simulink model "COHERENT_DEMODULATOR"  (R2021b)
settings: Solver=VariableStepAuto  StartTime=0.0  StopTime=0.002  RelTol=1e-3
libraries: simulink x3, commfilt2 x2, dspsigops x2, dspsrcs4 x2
settings Model: Creator=caccolillo  LastModifiedBy=caccolillo

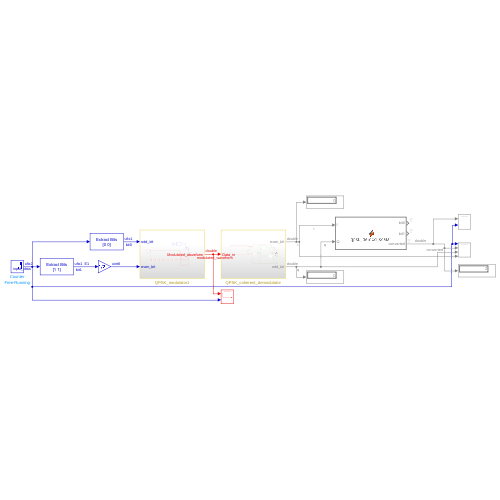
[thumbnail: Simulink's stored preview of the top-level diagram]
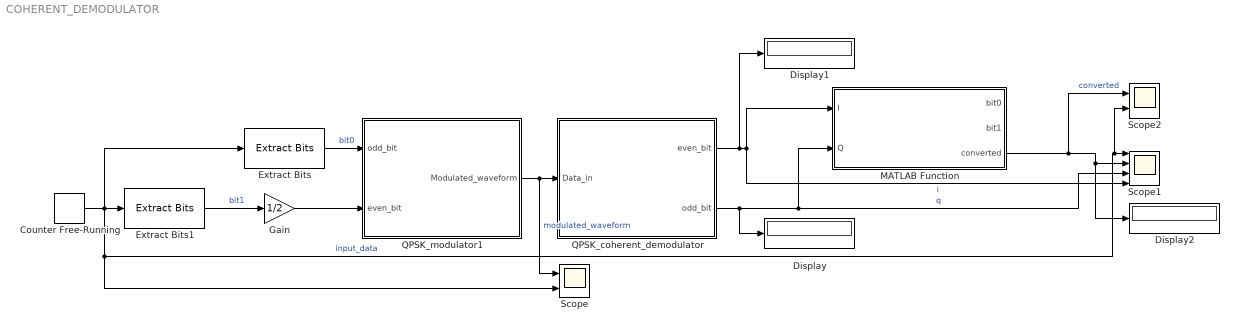
== system COHERENT_DEMODULATOR ==
  Counter Free-Running : simulink/Sources/Counter Free-Running  NumBits=2  tsamp=1/20000
  Display : Display
  Display1 : Display
  Display2 : Display
  Extract Bits : simulink/Logic and Bit Operations/Extract Bits  bitsToExtract=Range of bits  numBits=8  bitIdxRange=[0 0]  outScalingMode=Preserve fixed-point scaling
  Extract Bits1 : simulink/Logic and Bit Operations/Extract Bits  bitsToExtract=Range of bits  numBits=8  bitIdxRange=[1 1]  outScalingMode=Preserve fixed-point scaling
  Gain : Gain  Gain=1/2
  MATLAB Function : MATLAB Function  TreatAsAtomicUnit=on
  QPSK_coherent_demodulator : Subsystem
  QPSK_modulator1 : Subsystem
  Scope : Scope  NumInputPorts=2
  Scope1 : Scope  NumInputPorts=4
  Scope2 : Scope  NumInputPorts=2
  wires:
  QPSK_modulator1/1(Modulated_waveform) -> QPSK_coherent_demodulator/1(Data_in), Scope/1  "modulated_waveform"
  Counter Free-Running/1 -> Scope2/2, Scope1/1, Scope/2, Extract Bits/1, Extract Bits1/1  "input_data"
  QPSK_coherent_demodulator/2(odd_bit) -> MATLAB Function/2(Q), Scope1/3, Display/1  "q"
  QPSK_coherent_demodulator/1(even_bit) -> MATLAB Function/1(I), Scope1/4, Display1/1  "i"
  Gain/1 -> QPSK_modulator1/2(even_bit)
  MATLAB Function/3(converted) -> Scope2/1, Display2/1, Scope1/2  "converted"
  Extract Bits/1 -> QPSK_modulator1/1(odd_bit)  "bit0"
  Extract Bits1/1 -> Gain/1  "bit1"

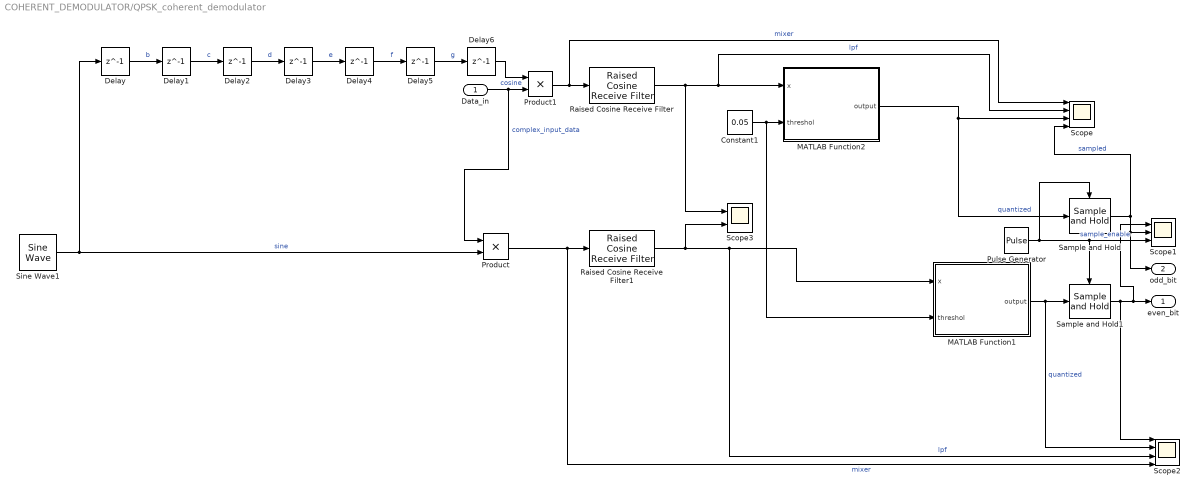
== system COHERENT_DEMODULATOR/QPSK_coherent_demodulator ==
  Data_in : Inport
  Constant1 : Constant  Value=0.05
  Delay{,1..6} (7 alike) : Delay  DelayLength=1  InitialCondition=0
  MATLAB Function1 : MATLAB Function  TreatAsAtomicUnit=on
  MATLAB Function2 : MATLAB Function  TreatAsAtomicUnit=on
  Product : Product
  Product1 : Product
  Pulse Generator : DiscretePulseGenerator  PulseType=Time based  Period=1/20000  PulseWidth=5
  Raised Cosine Receive Filter : commfilt2/Raised Cosine Receive Filter  filtType=Square root  R=0.2  filtSpan=10  N=10  downFactor=2  downOffset=0  filterGain=1  RateOptions=Allow multirate processing  framing=Mute  checkCoeff=off  variableName=rcRxFilt  currentFiltSpan=10  D=5  inputOffset=0  sampMode=Mute  saveAsFlag=0  rateMode=Downsampling  checkGain=Normalized  launchFVT=on  roundingMode=Floor  overflowMode=off  coeffDataTypeStr=Inherit: Same word length as input  coeffMin=[]  coeffMax=[]  coeffLastDataTypeStr=Inherit: Same word length as input  accumDataTypeStr=Inherit: Same as product output  accumLastDataTypeStr=Inherit: Same as product output  outputDataTypeStr=Inherit: Same as accumulator  outputMin=[]  outputMax=[]  outputLastDataTypeStr=Inherit: Same as accumulator
  Raised Cosine Receive Filter1 : commfilt2/Raised Cosine Receive Filter  filtType=Square root  R=0.2  filtSpan=10  N=10  downFactor=2  downOffset=0  filterGain=1  RateOptions=Allow multirate processing  framing=Mute  checkCoeff=off  variableName=rcRxFilt1  currentFiltSpan=10  D=5  inputOffset=0  sampMode=Mute  saveAsFlag=0  rateMode=Downsampling  checkGain=Normalized  launchFVT=on  roundingMode=Floor  overflowMode=off  coeffDataTypeStr=Inherit: Same word length as input  coeffMin=[]  coeffMax=[]  coeffLastDataTypeStr=Inherit: Same word length as input  accumDataTypeStr=Inherit: Same as product output  accumLastDataTypeStr=Inherit: Same as product output  outputDataTypeStr=Inherit: Same as accumulator  outputMin=[]  outputMax=[]  outputLastDataTypeStr=Inherit: Same as accumulator
  Sample and Hold : dspsigops/Sample and Hold  trig=Rising edge  initCond=0  latchinput=off
  Sample and Hold1 : dspsigops/Sample and Hold  trig=Rising edge  initCond=0  latchinput=off
  Scope : Scope  NumInputPorts=4
  Scope1 : Scope  NumInputPorts=3
  Scope2 : Scope  NumInputPorts=4
  Scope3 : Scope  NumInputPorts=2
  Sine Wave1 : dspsrcs4/Sine Wave  Amplitude=0.5  Frequency=20000  Phase=0  SampleMode=Discrete  OutComplex=Real  CompMethod=Table lookup  TableSize=Speed  SampleTime=1/200000  SamplesPerFrame=1  ResetState=Restart at time zero  OutputFrames=off  dataType=double  wordLen=16  udDataType=sfix(16)  fracBitsMode=Best precision  numFracBits=15  OutDataTypeStr=double  LastOutDataTypeStr=double
  even_bit : Outport
  odd_bit : Outport  Port=2
  wires:
  Data_in/1 -> Product1/2, Product/1  "complex_input_data"
  Product1/1 -> Raised Cosine Receive Filter/1, Scope/1  "mixer"
  Raised Cosine Receive Filter/1 -> Scope3/1, Scope/2, MATLAB Function2/1(x)  "lpf"
  Pulse Generator/1 -> Sample and Hold1/Trigger, Scope1/3, Sample and Hold/Trigger  "sample_enable"
  Product/1 -> Raised Cosine Receive Filter1/1, Scope2/4  "mixer"
  MATLAB Function1/1(output) -> Scope2/2, Sample and Hold1/1  "quantized"
  Sine Wave1/1 -> Delay/1, Product/2  "sine"
  Delay2/1 -> Delay3/1  "d"
  Delay3/1 -> Delay4/1  "e"
  Delay/1 -> Delay1/1  "b"
  Sample and Hold/1 -> Scope1/2, odd_bit/1, Scope/4  "sampled"
  Delay5/1 -> Delay6/1  "g"
  Sample and Hold1/1 -> Scope2/1, Scope1/1, even_bit/1
  Delay1/1 -> Delay2/1  "c"
  Delay6/1 -> Product1/1  "cosine"
  Raised Cosine Receive Filter1/1 -> Scope3/2, Scope2/3, MATLAB Function1/1(x)  "lpf"
  Delay4/1 -> Delay5/1  "f"
  Constant1/1 -> MATLAB Function1/2(threshol), MATLAB Function2/2(threshol)
  MATLAB Function2/1(output) -> Scope/3, Sample and Hold/1  "quantized"

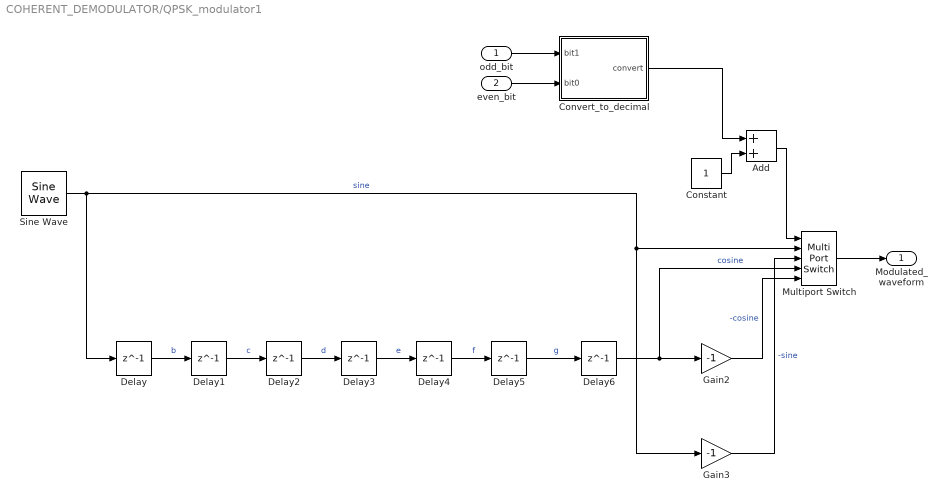
== system COHERENT_DEMODULATOR/QPSK_modulator1 ==
  odd_bit : Inport
  even_bit : Inport  Port=2
  Add : Sum
  Constant : Constant
  Convert_to_decimal : Subsystem
  Delay{,1..6} (7 alike) : Delay  DelayLength=1  InitialCondition=0
  Gain2 : Gain  Gain=-1
  Gain3 : Gain  Gain=-1
  Multiport Switch : MultiPortSwitch  Inputs=4
  Sine Wave : dspsrcs4/Sine Wave  Amplitude=1  Frequency=20000  Phase=0  SampleMode=Discrete  OutComplex=Real  CompMethod=Table lookup  TableSize=Speed  SampleTime=1/200000  SamplesPerFrame=1  ResetState=Restart at time zero  OutputFrames=off  dataType=double  wordLen=16  udDataType=sfix(16)  fracBitsMode=Best precision  numFracBits=15  OutDataTypeStr=double  LastOutDataTypeStr=double
  Modulated_waveform : Outport
  wires:
  Gain3/1 -> Multiport Switch/3  "-sine"
  Sine Wave/1 -> Multiport Switch/2, Gain3/1, Delay/1  "sine"
  Delay/1 -> Delay1/1  "b"
  Delay1/1 -> Delay2/1  "c"
  Delay6/1 -> Multiport Switch/4, Gain2/1  "cosine"
  Multiport Switch/1 -> Modulated_waveform/1
  Delay3/1 -> Delay4/1  "e"
  Gain2/1 -> Multiport Switch/5  "-cosine"
  Delay4/1 -> Delay5/1  "f"
  odd_bit/1 -> Convert_to_decimal/1(bit1)
  Delay2/1 -> Delay3/1  "d"
  Convert_to_decimal/1(convert) -> Add/1
  Constant/1 -> Add/2
  Add/1 -> Multiport Switch/1
  even_bit/1 -> Convert_to_decimal/2(bit0)
  Delay5/1 -> Delay6/1  "g"

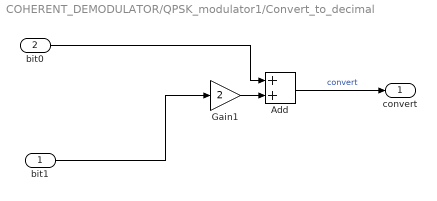
== system COHERENT_DEMODULATOR/QPSK_modulator1/Convert_to_decimal ==
  bit1 : Inport
  bit0 : Inport  Port=2
  Add : Sum
  Gain1 : Gain  Gain=2
  convert : Outport
  wires:
  bit1/1 -> Gain1/1
  bit0/1 -> Add/1
  Add/1 -> convert/1  "convert"
  Gain1/1 -> Add/2

== matlab function COHERENT_DEMODULATOR/QPSK_coherent_demodulator/MATLAB Function1 ==
  data: x input; output output; threshol input
function output = discretize_input(x,threshol)
    if x > threshol
        output = 1;
    else
        output = 0;
    end
end

== matlab function COHERENT_DEMODULATOR/QPSK_coherent_demodulator/MATLAB Function2 ==
  data: x input; output output; threshol input
function output = discretize_input(x,threshol)
    if x > threshol
        output = 1;
    else
        output = 0;
    end
end

== matlab function COHERENT_DEMODULATOR/MATLAB Function ==
  data: bit0 output; I input; bit1 output; Q input; converted output
function [bit0, bit1,converted] = qpsk_demod_scalar(I, Q)
%QPSK_DEMOD_SCALAR Demodulates one QPSK symbol (scalar I/Q) into two bits.
% Inputs:
%   I - In-phase component (scalar)
%   Q - Quadrature component (scalar)
% Outputs:
%   bit1 - First bit (MSB)
%   bit2 - Second bit (LSB)

    % QPSK Gray demapping
    if I == 1 && Q == 1
        bit0 = 0; bit1 = 0;
        converted = 0;
    elseif I == 0 && Q == 1
        bit0 = 0; bit1 = 1;
        converted = 1;
    elseif I == 0 && Q == 0
        bit0 = 0; bit1 = 1;
        converted = 2;
    elseif I == 1 && Q == 0
        bit0 = 1; bit1 = 1;
        converted = 3;
    else
        % Edge case: I or Q == 0 (treat as 0)
        bit0 = 0;
        bit1 = 0;
        converted = 0;
    end
end
